simulink subsystem "SchlittenPendel"  (R2020a)
settings: Solver=VariableStepAuto  StartTime=0.0  StopTime=10.0  RelTol=1e-3
model mask{params=[]}
undefined symbols (not defined in the file or in its folder): simparams
Description:
  | Modell des Schlitten-Doppelpendel-Systems
  | Eingang: Kraft
  | Ausgang: Zustände (6), Ausgänge (3)
settings Model: Creator=Tobias  LastModifiedBy=Frederik

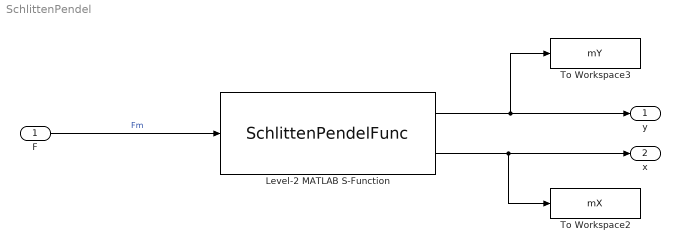
== system SchlittenPendel ==
  F : Inport
  Level-2 MATLAB S-Function : M-S-Function  FunctionName=SchlittenPendelFunc  Parameters=params.x0 true
  To Workspace2 : ToWorkspace  VariableName=mX  SaveFormat=Timeseries  SampleTime=simparams.tows_ts
  To Workspace3 : ToWorkspace  VariableName=mY  SaveFormat=Timeseries  SampleTime=simparams.tows_ts
      settings: Save2DSignal=2-D array (concatenate along first dimension)
  y : Outport
  x : Outport  Port=2
  wires:
  F/1 -> Level-2 MATLAB S-Function/1  "Fm"
  Level-2 MATLAB S-Function/1 -> y/1, To Workspace3/1
  Level-2 MATLAB S-Function/2 -> To Workspace2/1, x/1
